simulink model "gru_FL_test"  (R2020a)
settings: Solver=FixedStepAuto  StartTime=0.0  StopTime=Inf  FixedStep=0.001  MaxStep=0.01  RelTol=1e-3
InitFcn:
  | init_gru
StopFcn:
  | %stop_gru
values from neighbouring files (symbols this model uses):
  centro = [points(1); points(2)]    [init_gru.m]
  dir_retta = [1; 0]    [init_gru.m]
  K1 = [1; 1; 1]    [init_gru.m]
  K2 = [0.5; 0.5; 0.5]    [init_gru.m]
  L_ddot_sat = Inf    (= inf)    [init_gru.m]
  L_dot_iniziale = 0    [init_gru.m]
  L_iniziale = z_b_iniziale/cos(theta_iniziale)    [init_gru.m]
  Lsofar = [Lsofar; sum(Lenghts)]    [init_gru.m]
  Ltot = sum(Lenghts)    [init_gru.m]
  n_p = length(points)    [init_gru.m]
  phi_dot_iniziale = 0    [init_gru.m]
  phi_iniziale = 30/180*pi    (= 0.523598775598)    [init_gru.m]
  s_finale = norm(traslazione,2)    [init_gru.m]
  theta_dot_iniziale = 0    [init_gru.m]
  theta_iniziale = 1e-2/180*pi    (= 0.000174532925199)    [init_gru.m]
  theta_rette = [theta_rette ; theta_rette(n_p-2)+pi]    [init_gru.m]
  v_r = v_rif    (= 1)    [init_gru.m]
  x_b_iniziale = 0    [init_gru.m]
  x_t_ddot_sat = Inf    (= inf)    [init_gru.m]
  x_t_dot_iniziale = 0    [init_gru.m]
  x_t_iniziale = x_b_iniziale - L_iniziale * sin(theta_iniziale) * sin(phi_iniziale)    [init_gru.m]
  xp = points(:,1)    [init_gru.m]
  y_b_iniziale = 0    [init_gru.m]
  y_t_ddot_sat = Inf    (= inf)    [init_gru.m]
  y_t_dot_iniziale = 0    [init_gru.m]
  y_t_iniziale = y_b_iniziale - L_iniziale * sin(theta_iniziale) * cos(phi_iniziale)    [init_gru.m]
  yp = points(:,2)    [init_gru.m]
  z_b_iniziale = 2    [init_gru.m]
undefined symbols (not defined in the file or in its folder): indexclot, Lsofarclot, x_M_finale, x_M_iniziale, y_M_finale, y_M_iniziale
libraries: robotcorelib x2, simulink x1
settings Model: Creator=Andrea_Ferroni  LastModifiedBy=Francesco

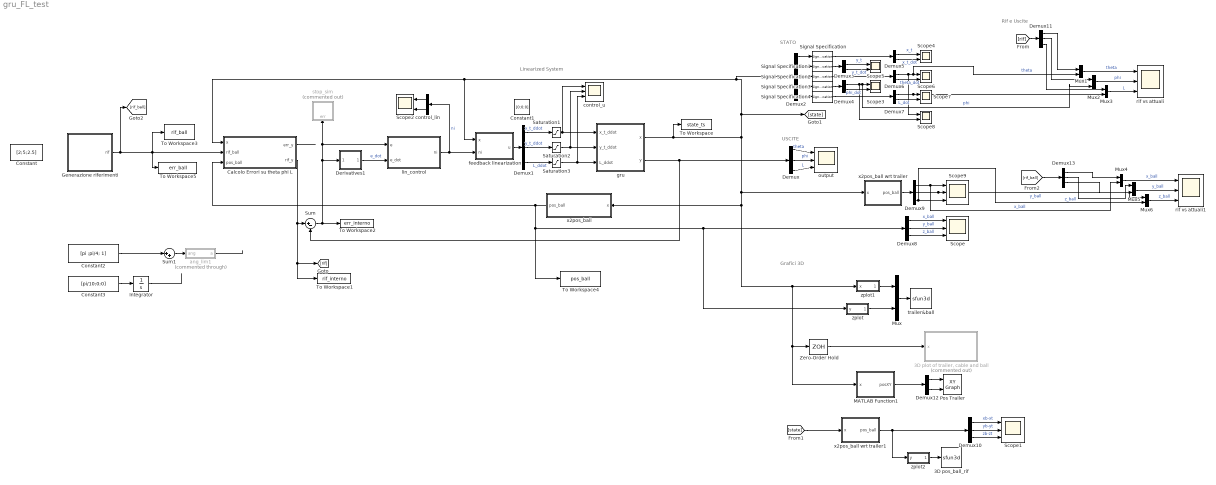
== system gru_FL_test ==
  note: Rif e Uscite
  note: Grafici 3D
  note: USCITE
  note: STATO
  note: Linearized System
  "3D plot of trailer, cable and ball" : MATLAB Function  Commented=on  TreatAsAtomicUnit=on
  3D pos_ball_rif : S-Function  LoadFcn=if exist('sfun3d','file'), sfun3d([],[],[],'LoadBlock'); end  FunctionName=sfun3d  Parameters=ax,T,np,cp,gd,ls,mk,mx,hd,tb  SFunctionDeploymentMode=off  EnableBusSupport=off  mask(3D Graph){np=1, ax=[-50 50 -50 50 -3 3], mx=1e4, T=0.1, cp=[3 2 1], gd=on, hd=off, tb=off, ls=-, mk=none}
      mask prompts: np "Number of moving points (lines)"; ax "Range: [xmin xmax  ymin ymax zmin zmax]"; mx "Max number of points in each line"; T "Sampling Time"; cp "Camera position (use [0 0 1] for 2D XY view)"; gd "Grid (on|off)"; hd "HeadMarkers (on|off)"; tb "Toolbar (on|off)"; ls "LineStyle"; mk "LineMarker"
      mask help:
      | This block plots the position of several points in the XYZ space. The input contains the coordinates of all the points (x1,y1,z1,x2,y2,z2,...).
      | The number of moving points (lines), the XYZ ranges, sampling time, camera position, and grid (among other things) can be set as mask parameters.
      settings: CopyFcn=if exist('sfun3d','file'), sfun3d([],[],[],'CopyBlock'); end  DeleteFcn=if exist('sfun3d','file'), sfun3d([],[],[],'DeleteBlock'); end  NameChangeFcn=if exist('sfun3d','file'), sfun3d([],[],[],'NameChange'); end
      mask Help:
      | This block plots the position of several points in the XYZ space. The input contains the coordinates of all the points (x1,y1,z1,x2,y2,z2,...).
      | The number of moving points (lines), the XYZ ranges, sampling time, camera position, and grid (among other things) can be set as mask parameters.
      mask TypeOptions ls: - | -- | : | -. | none
      mask TypeOptions mk: none | . | + | o | * | x | square | diamond | v | ^ | > | < | pentagram | hexagram
      mask Display: plot([.05 .95 .95 .05 .05],[.45 .45 .95 .95 .45], 0.5+cos(0:0.1:2*pi)*0.3,0.7+sin(0:0.1:2*pi)*0.2)
  Calcolo Errori su theta phi L : MATLAB Function  TreatAsAtomicUnit=on
  Constant : Constant  Value=[2;5;2.5]
  Constant1 : Constant  Value=[0;0;0]
  Constant2 : Constant  Value=[pi ;pi/4; 1]
  Constant3 : Constant  Value=[pi/10;0;0]
  Demux{,1,8..11,13} (7 alike) : Demux  Outputs=3
  Demux{3..7,12} (6 alike) : Demux  Outputs=2
  Demux2 : Demux  Outputs=5
  Derivatives1 : Subsystem
  Generazione riferimenti : Subsystem  Variant=on
  Integrator : Integrator
  MATLAB Function1 : MATLAB Function  TreatAsAtomicUnit=on
  Mux{,1..6} (7 alike) : Mux  Inputs=2
  Pos Trailer : simulink/Sinks/XY Graph  xmin=-100  xmax=100  ymin=-100  ymax=100  st=-1
  Saturation1 : Saturate  UpperLimit=x_t_ddot_sat  LowerLimit=-x_t_ddot_sat
  Saturation2 : Saturate  UpperLimit=y_t_ddot_sat  LowerLimit=-y_t_ddot_sat
  Saturation3 : Saturate  UpperLimit=L_ddot_sat  LowerLimit=-L_ddot_sat
  Scope : Scope  NumInputPorts=3
  Scope1 : Scope  NumInputPorts=3
  Scope{2..8} (7 alike) : Scope  NumInputPorts=2
  Scope9 : Scope  NumInputPorts=3
  Signal Specification{,1..4} (5 alike) : SignalSpecification  Dimensions=[2]
  Sum : Sum  Inputs=|+-
  Sum1 : Sum  Inputs=|++
  To Workspace : ToWorkspace  VariableName=state_ts  SaveFormat=Timeseries  SampleTime=-1
  To Workspace1 : ToWorkspace  VariableName=rif_interno  SaveFormat=Timeseries  SampleTime=-1
  To Workspace2 : ToWorkspace  VariableName=err_interno  SaveFormat=Timeseries  SampleTime=-1
  To Workspace3 : ToWorkspace  VariableName=rif_ball  SaveFormat=Timeseries  SampleTime=-1
  To Workspace4 : ToWorkspace  VariableName=pos_ball  SaveFormat=Timeseries  SampleTime=-1
  To Workspace5 : ToWorkspace  VariableName=err_ball  SaveFormat=Timeseries  SampleTime=-1
  Zero-Order Hold : ZeroOrderHold  SampleTime=1/10
  ang_lim1 : MATLAB Function  Commented=through  TreatAsAtomicUnit=on
  control_lin : Demux  Outputs=2
  control_u : Scope  NumInputPorts=3
  feedback linearization : MATLAB Function  TreatAsAtomicUnit=on
  gru : Subsystem
      mask Display: image('$imagefile'); % Use "Edit Image" on toolstrip to change.
  lin_control : MATLAB Function  TreatAsAtomicUnit=on
  output : Scope  NumInputPorts=3
  rif vs attuali : Scope  NumInputPorts=3
  rif vs attuali1 : Scope  NumInputPorts=3
  stop_sim : Subsystem  Commented=on
  trailer&ball : S-Function  LoadFcn=if exist('sfun3d','file'), sfun3d([],[],[],'LoadBlock'); end  FunctionName=sfun3d  Parameters=ax,T,np,cp,gd,ls,mk,mx,hd,tb  SFunctionDeploymentMode=off  EnableBusSupport=off  mask(3D Graph){np=2, ax=[-50 50 -50 50 -3 3], mx=1e4, T=0.1, cp=[3 2 1], gd=on, hd=off, tb=off, ls=-, mk=none}
      mask prompts: np "Number of moving points (lines)"; ax "Range: [xmin xmax  ymin ymax zmin zmax]"; mx "Max number of points in each line"; T "Sampling Time"; cp "Camera position (use [0 0 1] for 2D XY view)"; gd "Grid (on|off)"; hd "HeadMarkers (on|off)"; tb "Toolbar (on|off)"; ls "LineStyle"; mk "LineMarker"
      mask help:
      | This block plots the position of several points in the XYZ space. The input contains the coordinates of all the points (x1,y1,z1,x2,y2,z2,...).
      | The number of moving points (lines), the XYZ ranges, sampling time, camera position, and grid (among other things) can be set as mask parameters.
      settings: CopyFcn=if exist('sfun3d','file'), sfun3d([],[],[],'CopyBlock'); end  DeleteFcn=if exist('sfun3d','file'), sfun3d([],[],[],'DeleteBlock'); end  NameChangeFcn=if exist('sfun3d','file'), sfun3d([],[],[],'NameChange'); end
      mask Help:
      | This block plots the position of several points in the XYZ space. The input contains the coordinates of all the points (x1,y1,z1,x2,y2,z2,...).
      | The number of moving points (lines), the XYZ ranges, sampling time, camera position, and grid (among other things) can be set as mask parameters.
      mask TypeOptions ls: - | -- | : | -. | none
      mask TypeOptions mk: none | . | + | o | * | x | square | diamond | v | ^ | > | < | pentagram | hexagram
      mask Display: plot([.05 .95 .95 .05 .05],[.45 .45 .95 .95 .45], 0.5+cos(0:0.1:2*pi)*0.3,0.7+sin(0:0.1:2*pi)*0.2)
  x2pos_ball : MATLAB Function  TreatAsAtomicUnit=on
  x2pos_ball wrt trailer : MATLAB Function  TreatAsAtomicUnit=on
  x2pos_ball wrt trailer1 : MATLAB Function  TreatAsAtomicUnit=on
  zplot : MATLAB Function  TreatAsAtomicUnit=on
  zplot1 : MATLAB Function  TreatAsAtomicUnit=on
  zplot2 : MATLAB Function  TreatAsAtomicUnit=on
  wires:
  gru/2(y) -> Sum/2, Demux/1
  lin_control/1(ni) -> control_lin/1, feedback linearization/2(ni)  "ni"
  Derivatives1/1(Out1) -> lin_control/2(e_dot)  "e_dot"
  Demux1/1 -> Saturation1/1  "x_t_ddot"
  Demux1/2 -> Saturation2/1  "y_t_ddot"
  control_lin/2 -> Scope2/2
  control_lin/1 -> Scope2/1
  Demux1/3 -> Saturation3/1  "L_ddot"
  Demux2/1 -> Signal Specification/1
  Demux2/2 -> Signal Specification1/1
  Signal Specification1/1 -> Demux3/1
  Demux2/3 -> Signal Specification2/1
  Demux2/4 -> Signal Specification3/1
  Demux2/5 -> Signal Specification4/1
  Demux3/1 -> Scope5/1  "y_t"
  Demux3/2 -> Scope5/2  "y_t_dot"
  Demux4/1 -> Mux2/2, Scope3/1, Scope8/2  "phi"
  Demux4/2 -> Scope3/2  "phi_dot"
  Signal Specification3/1 -> Demux4/1
  Demux5/1 -> Scope4/1  "x_t"
  Demux5/2 -> Scope4/2  "x_t_dot"
  Signal Specification/1 -> Demux5/1
  Demux6/1 -> Scope8/1, Mux1/2, Scope6/1  "theta"
  Demux6/2 -> Scope6/2  "theta_dot"
  Signal Specification2/1 -> Demux6/1
  Demux7/1 -> Mux3/2, Scope7/1
  Demux7/2 -> Scope7/2  "L_dot"
  Signal Specification4/1 -> Demux7/1
  zplot/1(y_new) -> Mux/2
  Mux/1 -> trailer&ball/1
  zplot1/1(trailer_graph) -> Mux/1
  feedback linearization/1(u) -> Demux1/1
  Demux8/3 -> Scope/3  "z_ball"
  Demux8/2 -> Scope/2  "y_ball"
  Demux8/1 -> Scope/1  "x_ball"
  x2pos_ball wrt trailer/1(pos_ball) -> Demux9/1
  x2pos_ball/1(pos_ball) -> zplot/1(y), Demux8/1, To Workspace4/1, Calcolo Errori su theta phi L/3(pos_ball)
  Demux9/1 -> Mux4/2, Scope9/1  "x_ball"
  Demux9/2 -> Mux5/2, Scope9/2  "y_ball"
  Demux9/3 -> Mux6/2, Scope9/3  "z_ball"
  Sum/1 -> stop_sim/1(err), lin_control/1(e), Derivatives1/1(In1), To Workspace2/1
  Demux/1 -> output/1  "theta"
  Demux/2 -> output/2  "phi"
  Demux/3 -> output/3  "L"
  Demux10/3 -> Scope1/3  "zb-zt"
  Demux10/1 -> Scope1/1  "xb-xt"
  Demux10/2 -> Scope1/2  "yb-yt"
  x2pos_ball wrt trailer1/1(pos_ball) -> zplot2/1(y), Demux10/1
  zplot2/1(y_new) -> 3D pos_ball_rif/1
  Demux11/2 -> Mux2/1
  Demux11/1 -> Mux1/1
  Mux3/1 -> rif vs attuali/3  "L"
  Mux2/1 -> rif vs attuali/2  "phi"
  MATLAB Function1/1(posXY) -> Demux12/1
  Demux12/1 -> Pos Trailer/1
  Demux12/2 -> Pos Trailer/2
  Zero-Order Hold/1 -> "3D plot of trailer, cable and ball"/1(x)
  Saturation1/1 -> control_u/1, gru/1(x_t_ddot)
  Saturation2/1 -> gru/2(y_t_ddot), control_u/2
  Saturation3/1 -> control_u/3, gru/3(L_ddot)
  Demux11/3 -> Mux3/1
  Mux1/1 -> rif vs attuali/1  "theta"
  [rif] -> Demux11/1
  gru/1(x) -> Zero-Order Hold/1, MATLAB Function1/1(x), zplot1/1(x), x2pos_ball/1(x), x2pos_ball wrt trailer/1(x), feedback linearization/1(x), Calcolo Errori su theta phi L/1(x), Demux2/1, [state], To Workspace/1
  [state] -> x2pos_ball wrt trailer1/1(x)
  Sum1/1 -> ang_lim1/1(ang)
  Constant2/1 -> Sum1/1
  Constant3/1 -> Integrator/1
  Integrator/1 -> ?
  Calcolo Errori su theta phi L/1(err_y) -> ?
  Generazione riferimenti/1(rif) -> [rif_ball], To Workspace5/1, To Workspace3/1, Calcolo Errori su theta phi L/2(rif_ball)
  Calcolo Errori su theta phi L/2(rif_y) -> To Workspace1/1, [rif], Sum/1
  ang_lim1/1(a) -> ?
  Mux6/1 -> rif vs attuali1/3  "z_ball"
  Mux4/1 -> rif vs attuali1/1  "x_ball"
  Mux5/1 -> rif vs attuali1/2  "y_ball"
  [rif_ball] -> Demux13/1
  Demux13/1 -> Mux4/1
  Demux13/2 -> Mux5/1
  Demux13/3 -> Mux6/1

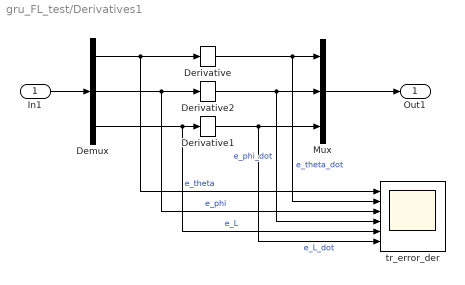
== system gru_FL_test/Derivatives1 ==
  In1 : Inport
  Demux : Demux  Outputs=3
  Derivative : Derivative  CoefficientInTFapproximation=1e10
  Derivative1 : Derivative  CoefficientInTFapproximation=1e10
  Derivative2 : Derivative  CoefficientInTFapproximation=1e10
  Mux : Mux  Inputs=3
  tr_error_der : Scope  NumInputPorts=6
  Out1 : Outport
  wires:
  Mux/1 -> Out1/1
  Demux/2 -> tr_error_der/3, Derivative2/1  "e_phi"
  Derivative/1 -> tr_error_der/2, Mux/1  "e_theta_dot"
  Demux/1 -> tr_error_der/1, Derivative/1  "e_theta"
  In1/1 -> Demux/1
  Derivative2/1 -> tr_error_der/4, Mux/2  "e_phi_dot"
  Demux/3 -> tr_error_der/5, Derivative1/1  "e_L"
  Derivative1/1 -> tr_error_der/6, Mux/3  "e_L_dot"

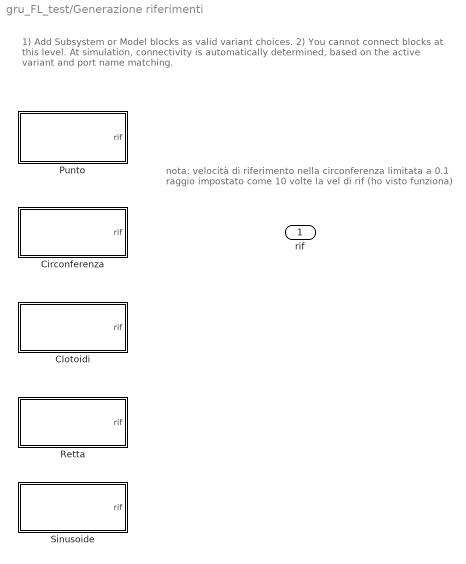
== system gru_FL_test/Generazione riferimenti ==
  note: nota:
      | velocità di riferimento nella circonferenza limitata a 0.1
      | raggio impostato come 10 volte la vel di rif (ho visto funziona)
  note: 1) Add Subsystem or Model blocks as valid variant choices.
      | 2) You cannot connect blocks at this level. At simulation, connectivity is automatically
      | determined, based on the active variant and port name matching.
  Circonferenza : Subsystem  VariantControl=Circonferenza
  Clotoidi : Subsystem  VariantControl=Clotoidi
  Punto : Subsystem  VariantControl=Punto
  Retta : Subsystem  VariantControl=Retta
  Sinusoide : Subsystem  VariantControl=Sinusoide
  rif : Outport

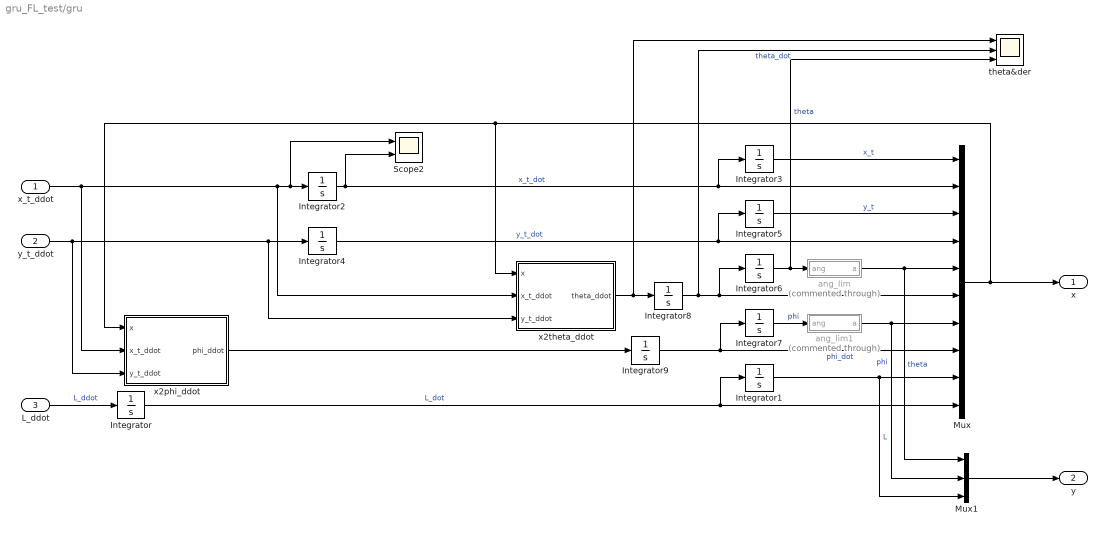
== system gru_FL_test/gru ==
  x_t_ddot : Inport
  y_t_ddot : Inport  Port=2
  L_ddot : Inport  Port=3
  Integrator : Integrator  InitialCondition=L_dot_iniziale
  Integrator1 : Integrator  InitialCondition=L_iniziale
  Integrator2 : Integrator  InitialCondition=x_t_dot_iniziale  UpperSaturationLimit=1e3  LowerSaturationLimit=-1e3
  Integrator3 : Integrator  InitialCondition=x_t_iniziale  LimitOutput=on  UpperSaturationLimit=10  LowerSaturationLimit=-10
  Integrator4 : Integrator  InitialCondition=y_t_dot_iniziale
  Integrator5 : Integrator  InitialCondition=y_t_iniziale  LimitOutput=on  UpperSaturationLimit=10  LowerSaturationLimit=-10
  Integrator6 : Integrator  InitialCondition=theta_iniziale
  Integrator7 : Integrator  InitialCondition=phi_iniziale
  Integrator8 : Integrator  InitialCondition=theta_dot_iniziale
  Integrator9 : Integrator  InitialCondition=phi_dot_iniziale
  Mux : Mux  Inputs=10
  Mux1 : Mux  Inputs=3
  Scope2 : Scope  NumInputPorts=2
  ang_lim : MATLAB Function  Commented=through  TreatAsAtomicUnit=on
  ang_lim1 : MATLAB Function  Commented=through  TreatAsAtomicUnit=on
  theta&der : Scope  NumInputPorts=3
  x2phi_ddot : MATLAB Function  TreatAsAtomicUnit=on
  x2theta_ddot : MATLAB Function  TreatAsAtomicUnit=on
  x : Outport
  y : Outport  Port=2
  wires:
  Integrator3/1 -> Mux/1  "x_t"
  Integrator2/1 -> Scope2/2, Integrator3/1, Mux/2  "x_t_dot"
  Integrator5/1 -> Mux/3  "y_t"
  Integrator4/1 -> Integrator5/1, Mux/4  "y_t_dot"
  Integrator6/1 -> theta&der/3, ang_lim/1(ang)  "theta"
  Integrator8/1 -> theta&der/2, Integrator6/1, Mux/6  "theta_dot"
  Integrator7/1 -> ang_lim1/1(ang)  "phi"
  Integrator9/1 -> Integrator7/1, Mux/8  "phi_dot"
  Integrator1/1 -> Mux1/3, Mux/9  "L"
  L_ddot/1 -> Integrator/1  "L_ddot"
  Integrator/1 -> Integrator1/1, Mux/10  "L_dot"
  x_t_ddot/1 -> x2theta_ddot/2(x_t_ddot), Scope2/1, Integrator2/1, x2phi_ddot/2(x_t_ddot)
  y_t_ddot/1 -> x2theta_ddot/3(y_t_ddot), Integrator4/1, x2phi_ddot/3(y_t_ddot)
  x2theta_ddot/1(theta_ddot) -> theta&der/1, Integrator8/1
  x2phi_ddot/1(phi_ddot) -> Integrator9/1
  Mux/1 -> x2phi_ddot/1(x), x2theta_ddot/1(x), x/1
  ang_lim/1(a) -> Mux1/1, Mux/5  "theta"
  ang_lim1/1(a) -> Mux1/2, Mux/7  "phi"
  Mux1/1 -> y/1

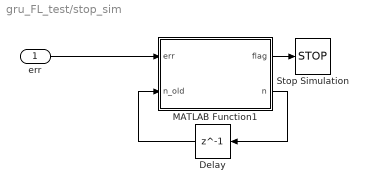
== system gru_FL_test/stop_sim ==
  err : Inport
  Delay : Delay  DelayLength=1
  MATLAB Function1 : MATLAB Function  TreatAsAtomicUnit=on
  Stop Simulation : Stop
  wires:
  MATLAB Function1/2(n) -> Delay/1
  MATLAB Function1/1(flag) -> Stop Simulation/1
  err/1 -> MATLAB Function1/1(err)
  Delay/1 -> MATLAB Function1/2(n_old)

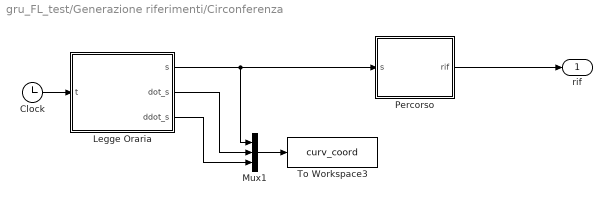
== system gru_FL_test/Generazione riferimenti/Circonferenza ==
  Clock : Clock
  Legge Oraria : MATLAB Function  TreatAsAtomicUnit=on
  Mux1 : Mux  Inputs=3
  Percorso : MATLAB Function  TreatAsAtomicUnit=on
  To Workspace3 : ToWorkspace  VariableName=curv_coord  SaveFormat=Timeseries  SampleTime=-1
  rif : Outport
  wires:
  Legge Oraria/2(dot_s) -> Mux1/2
  Clock/1 -> Legge Oraria/1(t)
  Mux1/1 -> To Workspace3/1
  Legge Oraria/3(ddot_s) -> Mux1/3
  Legge Oraria/1(s) -> Percorso/1(s), Mux1/1
  Percorso/1(rif) -> rif/1

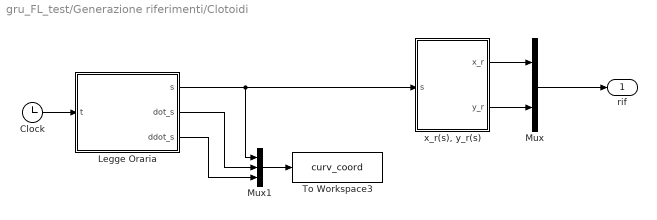
== system gru_FL_test/Generazione riferimenti/Clotoidi ==
  Clock : Clock
  Legge Oraria : MATLAB Function  TreatAsAtomicUnit=on
  Mux : Mux  Inputs=2
  Mux1 : Mux  Inputs=3
  To Workspace3 : ToWorkspace  VariableName=curv_coord  SaveFormat=Timeseries  SampleTime=-1
  "x_r(s), y_r(s)" : MATLAB Function  TreatAsAtomicUnit=on
  rif : Outport
  wires:
  Legge Oraria/1(s) -> Mux1/1, "x_r(s), y_r(s)"/1(s)
  Legge Oraria/2(dot_s) -> Mux1/2
  Clock/1 -> Legge Oraria/1(t)
  Legge Oraria/3(ddot_s) -> Mux1/3
  Mux1/1 -> To Workspace3/1
  "x_r(s), y_r(s)"/2(y_r) -> Mux/2
  "x_r(s), y_r(s)"/1(x_r) -> Mux/1
  Mux/1 -> rif/1

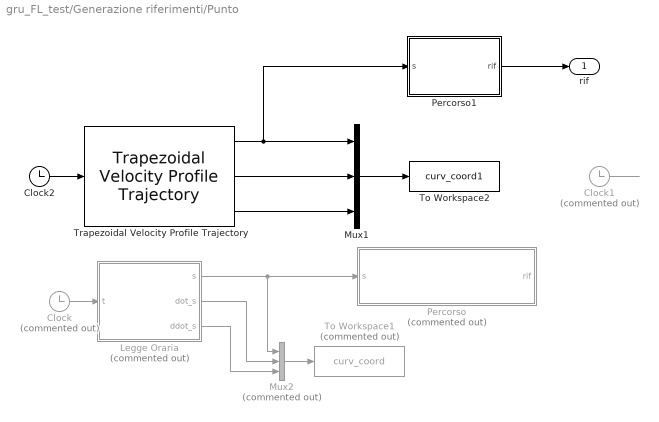
== system gru_FL_test/Generazione riferimenti/Punto ==
  Clock : Clock  Commented=on
  Clock1 : Clock  Commented=on
  Clock2 : Clock
  Legge Oraria : MATLAB Function  Commented=on  TreatAsAtomicUnit=on
  Mux1 : Mux  Inputs=3
  Mux2 : Mux  Commented=on  Inputs=3
  Percorso : MATLAB Function  Commented=on  TreatAsAtomicUnit=on
  Percorso1 : MATLAB Function  TreatAsAtomicUnit=on
  To Workspace1 : ToWorkspace  Commented=on  VariableName=curv_coord  SaveFormat=Timeseries  SampleTime=-1
  To Workspace2 : ToWorkspace  VariableName=curv_coord1  SaveFormat=Timeseries  SampleTime=-1
  Trapezoidal Velocity Profile Trajectory : robotcorelib/Trapezoidal Velocity Profile Trajectory  WaypointSource=Internal  Waypoints="[ 0,  s_finale]"  NumParams=2  Parameter1=Peak Velocity  Parameter2=Acceleration  ParameterSource=Internal  PeakVelocity=v_rif  Acceleration=a_rif  EndTime=[ 1; 1 ]  AccelTime=[ 1; 2 ]  SimulateUsing=Interpreted execution
      settings: SourceProductBaseCode=NV,RO,RR
  rif : Outport
  wires:
  Legge Oraria/2(dot_s) -> Mux2/2
  Clock/1 -> Legge Oraria/1(t)
  Mux2/1 -> To Workspace1/1
  Legge Oraria/3(ddot_s) -> Mux2/3
  Legge Oraria/1(s) -> Mux2/1, Percorso/1(s)
  Trapezoidal Velocity Profile Trajectory/1 -> Percorso1/1(s), Mux1/1
  Trapezoidal Velocity Profile Trajectory/2 -> Mux1/2
  Clock2/1 -> Trapezoidal Velocity Profile Trajectory/1
  Trapezoidal Velocity Profile Trajectory/3 -> Mux1/3
  Clock1/1 -> ?
  Mux1/1 -> To Workspace2/1
  Percorso1/1(rif) -> rif/1

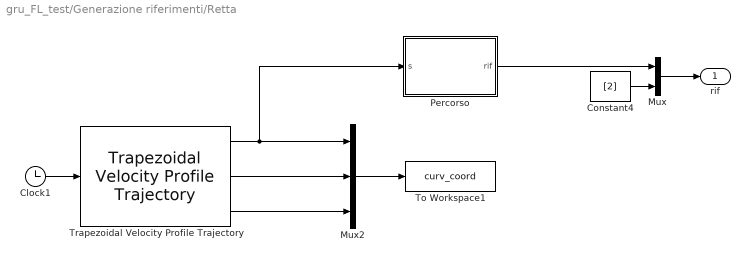
== system gru_FL_test/Generazione riferimenti/Retta ==
  Clock1 : Clock
  Constant4 : Constant  Value=[2]
  Mux : Mux  Inputs=2
  Mux2 : Mux  Inputs=3
  Percorso : MATLAB Function  TreatAsAtomicUnit=on
  To Workspace1 : ToWorkspace  VariableName=curv_coord  SaveFormat=Timeseries  SampleTime=-1
  Trapezoidal Velocity Profile Trajectory : robotcorelib/Trapezoidal Velocity Profile Trajectory  WaypointSource=Internal  Waypoints="[ 0,  1000]"  NumParams=2  Parameter1=Peak Velocity  Parameter2=Acceleration  ParameterSource=Internal  PeakVelocity=v_rif  Acceleration=a_rif  EndTime=[ 1; 1 ]  AccelTime=[ 1; 2 ]  SimulateUsing=Interpreted execution
      settings: SourceProductBaseCode=NV,RO,RR
  rif : Outport
  wires:
  Mux2/1 -> To Workspace1/1
  Clock1/1 -> Trapezoidal Velocity Profile Trajectory/1
  Trapezoidal Velocity Profile Trajectory/1 -> Percorso/1(s), Mux2/1
  Trapezoidal Velocity Profile Trajectory/2 -> Mux2/2
  Trapezoidal Velocity Profile Trajectory/3 -> Mux2/3
  Constant4/1 -> Mux/2
  Mux/1 -> rif/1
  Percorso/1(rif) -> Mux/1

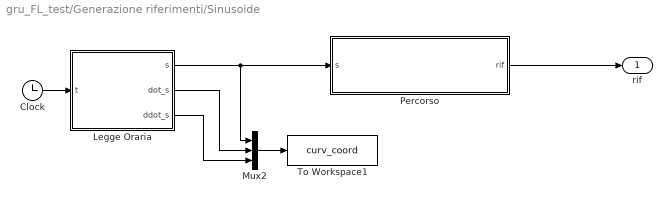
== system gru_FL_test/Generazione riferimenti/Sinusoide ==
  Clock : Clock
  Legge Oraria : MATLAB Function  TreatAsAtomicUnit=on
  Mux2 : Mux  Inputs=3
  Percorso : MATLAB Function  TreatAsAtomicUnit=on
  To Workspace1 : ToWorkspace  VariableName=curv_coord  SaveFormat=Timeseries  SampleTime=-1
  rif : Outport
  wires:
  Legge Oraria/2(dot_s) -> Mux2/2
  Clock/1 -> Legge Oraria/1(t)
  Mux2/1 -> To Workspace1/1
  Legge Oraria/3(ddot_s) -> Mux2/3
  Legge Oraria/1(s) -> Mux2/1, Percorso/1(s)
  Percorso/1(rif) -> rif/1

== matlab function gru_FL_test/gru/x2phi_ddot ==
  data: x input; phi_ddot output; x_t_ddot input; y_t_ddot input
function phi_ddot = fcn(x, x_t_ddot, y_t_ddot)
	
	theta		= x(5);
	theta_dot	= x(6);
	phi			= x(7);
	phi_dot		= x(8);
	L			= x(9);
	L_dot		= x(10);
	
phi_ddot = -2*(L_dot/L)*phi_dot-2*phi_dot*theta_dot*cot(theta) + (-cos(phi)/(sin(theta)*L))*x_t_ddot + (sin(phi)/(sin(theta)*L))*y_t_ddot;

== matlab function gru_FL_test/Generazione riferimenti/Circonferenza/Legge Oraria ==
  data: t input; s output; v_rif parameter; dot_s output; ddot_s output
function [s, dot_s, ddot_s]  = legge_oraria(t, v_rif)
%#codegen PEPO

s = v_rif*t;
dot_s = v_rif;
ddot_s = 0.0;


end

== matlab function gru_FL_test/Generazione riferimenti/Circonferenza/Percorso ==
  data: s input; rif output; centro parameter; v_r parameter
function rif = percorso(s, centro, v_r)

r = 10*v_r;  % 1
theta_circ = s/r;

if theta_circ >=  3*2*pi % dopotre giri ti fermi
	theta_circ = 3*2*pi;
end

rif = centro + r*[cos(theta_circ);sin(theta_circ)];		% circonferenza

end

== matlab function gru_FL_test/Generazione riferimenti/Retta/Percorso ==
  data: s input; rif output; dir_retta parameter; x_b_iniziale parameter; y_b_iniziale parameter
function rif  = retta(s, dir_retta, x_b_iniziale, y_b_iniziale)

rif = [x_b_iniziale;y_b_iniziale] + s * dir_retta;


end

== matlab function gru_FL_test/Generazione riferimenti/Clotoidi/x_r(s), y_r(s) ==
  data: s input; x_r output size=1; y_r output size=1; indexclot parameter; theta_rette parameter; yp parameter; xp parameter; Lsofar parameter; n_p parameter; Lsofarclot parameter; Ltot parameter
function [x_r,y_r] = percorso(s, indexclot, theta_rette, yp, xp, ...
										Lsofar, n_p, Lsofarclot, Ltot)
									
coder.extrinsic('pointsOnClothoid')
% fine percorso
if s >= Ltot
	s = Ltot; % cosi` da plottare l'ultimo punto
end

ntratto=0;
	XYS = [0; 0]; %definito prima

	%Parte per capire in che tratto sono
	if s < Lsofar(1)
		ntratto=1;
	else
		for ii=2:(n_p-1)
			if s>=Lsofar(ii-1) && s<=Lsofar(ii)
				ntratto=ii;
			end
		end
	end	

		%calcolo delle coordinate x e y riferite a s e a ntratto
	if mod(ntratto,2)==1            %tratti dispari - rette
		if ntratto==1
			XYS=[xp(ntratto)+cos(theta_rette(ntratto))*(s); ...
				yp(ntratto)+sin(theta_rette(ntratto))*(s)];
		else
			srel=s-Lsofar(ntratto-1);
			XYS=[	xp(ntratto)	+ cos(theta_rette(ntratto))	* srel; ...
					yp(ntratto)	+ sin(theta_rette(ntratto))	* srel];
		end 

	elseif mod(ntratto,2)==0	%tratti pari - clotoidi
		srel=s-Lsofar(ntratto-1);

		if srel<=Lsofarclot(ntratto/2).Lclot(1)
			XYS = double(pointsOnClothoid( indexclot(ntratto/2).clot.S0, srel ));

		elseif srel>Lsofarclot(ntratto/2).Lclot(1) & srel<=Lsofarclot(ntratto/2).Lclot(2)
			XYS = double(pointsOnClothoid( indexclot(ntratto/2).clot.SM, srel- indexclot(ntratto/2).clot.S0.L ));

		elseif srel>Lsofarclot(ntratto/2).Lclot(2)
			XYS = double(pointsOnClothoid( indexclot(ntratto/2).clot.S1, srel- indexclot(ntratto/2).clot.S0.L - indexclot(ntratto/2).clot.SM.L ));
		end

		%XYS = double(pointsOnClothoid( indexclot(ntratto/2).clot, s-Lsofar(ntratto-1) ));
	end

	x_r = XYS(1);
	y_r = XYS(2);
%--------------------------------------------------
% end function
end

== matlab function gru_FL_test/Generazione riferimenti/Sinusoide/Legge Oraria ==
  data: t input; s output; v_rif parameter; dot_s output; ddot_s output
function [s, dot_s, ddot_s]  = legge_oraria(t, v_rif)
%#codegen PEPO

s = v_rif*t;
dot_s = v_rif;
ddot_s = 0.0;


end

== matlab function gru_FL_test/Generazione riferimenti/Sinusoide/Percorso ==
  data: s input; rif output; dir_retta parameter
function rif  = retta(s, dir_retta)

r = 5;
theta_circ = s/r;

% if theta_circ >=  3*2*pi % dopotre giri ti fermi
% 	theta_circ = 3*2*pi;
% end

rif = dir_retta * s + r*[0; sin(theta_circ)];	% circonferenza

end

== matlab function gru_FL_test/x2pos_ball ==
  data: x input; pos_ball output; z_t parameter
function pos_ball = fcn(x, z_t)
	
	x_t		= x(1);
	y_t		= x(3);
	theta	= x(5);
	phi		= x(7);
	L		= x(9);
	
pos_ball = [x_t + L*sin(theta)*sin(phi); ...
			y_t + L*sin(theta)*cos(phi);...
			z_t + L*cos(theta)];

== matlab function gru_FL_test/x2pos_ball wrt trailer ==
  data: x input; pos_ball output
function pos_ball = fcn(x)
	
	theta	= x(5);
	phi		= x(7);
	L		= x(9);
	
pos_ball = [ L*sin(theta)*sin(phi); ...
			 L*sin(theta)*cos(phi);...
			 L*cos(theta)];

== matlab function gru_FL_test/gru/ang_lim ==
  data: ang input; a output
function a = ang_lim(ang)

	c = cos(ang);
	s = sin(ang);
	a = atan2(s, c);

end

== matlab function gru_FL_test/gru/ang_lim1 ==
  data: ang input; a output
function a = ang_lim(ang)

	c = cos(ang);
	s = sin(ang);
	a = atan2(s, c);

end

== matlab function gru_FL_test/zplot ==
  data: y input; y_new output
function y_new = fcn(y)

y_new	 = y;
y_new(3) = -y_new(3);

end

== matlab function gru_FL_test/zplot1 ==
  data: x input; trailer_graph output; z_t parameter
function trailer_graph = fcn(x, z_t)

	trailer_graph = [x(1); x(3); z_t];

end

== matlab function gru_FL_test/3D plot of trailer, cable and ball ==
  data: x input; z_t parameter
function gru_plot(x, z_t)

coder.extrinsic('plot3')
coder.extrinsic('text')
coder.extrinsic('num2str')

% get relevant signals
x_t		= x(1);
y_t		= x(3);
theta	= x(5);
phi		= x(7);
L		= x(9);

% get mass position
pos_ball = [ L*sin(theta)*sin(phi); ...
			 L*sin(theta)*cos(phi);...
			 -L*cos(theta)];

% figure
figure(1)
plot3(x_t, y_t, -z_t, 'bd', 'MarkerSize', 5)
hold on
plot3(pos_ball(1), pos_ball(2), pos_ball(3), 'ro', 'MarkerSize', 5)
plot3([x_t, pos_ball(1)], [y_t, pos_ball(2)], [-z_t, pos_ball(3)], 'k-', 'LineWidth', 2)
text(0,0,0,['theta ' num2str(theta/pi*180)])
grid on
view([45 10])
xlim([-50 50])
xlabel('X')
ylim([-50 50])
ylabel('Y')
zlim([-3 0.5])
zlabel('Z')
hold off
drawnow

end

== matlab function gru_FL_test/x2pos_ball wrt trailer1 ==
  data: x input; pos_ball output
function pos_ball = fcn(x)
	
	theta	= x(1);
	phi		= x(2);
	L		= x(3);
	
pos_ball = [ L*sin(theta)*sin(phi); ...
			 L*sin(theta)*cos(phi);...
			 L*cos(theta)];

== matlab function gru_FL_test/zplot2 ==
  data: y input; y_new output
function y_new = fcn(y)

y_new	 = y;
y_new(3) = -y_new(3);

end

== matlab function gru_FL_test/MATLAB Function1 ==
  data: x input; z_t parameter; posXY output
function posXY = pos_cart(x, z_t)

posXY = zeros(2,1);
% get relevant signals
posXY(1)		= x(1);
posXY(2)		= x(3);
%pos(3)		= z_t;

end

== matlab function gru_FL_test/ang_lim1 ==
  data: ang input; a output
function a = ang_lim(ang)

	c = cos(ang);
	s = sin(ang);
	a = atan2(s, c);

end

== matlab function gru_FL_test/Generazione riferimenti/Punto/Percorso1 ==
  data: s input; rif output; dir_retta parameter; x_b_iniziale parameter; y_b_iniziale parameter; z_b_iniziale parameter
function rif  = retta(s, dir_retta, x_b_iniziale, y_b_iniziale, z_b_iniziale)

rif = [x_b_iniziale; y_b_iniziale; z_b_iniziale] + s * dir_retta;


end

== matlab function gru_FL_test/Calcolo Errori su theta phi L ==
  data: err_y output; rif_y output; x input; rif_ball input; pos_ball input; z_t parameter
function [err_y, rif_y] = xyrif2err_y(x, rif_ball, pos_ball, z_t)

% Estraiamo i segnali utili
% attuali valori
x_t_now		= x(1);
y_t_now		= x(3);
theta_now	= x(5);
phi_now		= x(7);
L_now		= x(9);
pos_trailer = [x_t_now; y_t_now; z_t];


% err_palla
[theta_rif, phi_rif, L_rif] = pos2out(pos_trailer, rif_ball);
err_theta	= diffang(theta_now, theta_rif);	% theta_rif - theta_now
err_phi		= diffang(phi_now, phi_rif);		% phi_rif - phi_now
err_L		= L_rif - L_now;

% output of function
err_y = [err_theta; err_phi; err_L]; % theta - phi - L
rif_y = [theta_rif; phi_rif; L_rif];


end

%% Extra functions
function [theta, phi, L] = pos2out(pos_trailer, pos_ball)

xb = pos_ball(1);
yb = pos_ball(2);
zb = pos_ball(3);
xt = pos_trailer(1);
yt = pos_trailer(2);
zt = pos_trailer(3);

phi = atan2(xb-xt,yb-yt);

if phi < 1e-3
	theta = atan2(abs(yb-yt), zb-zt);
else
	theta = atan2(abs(xb-xt),(zb-zt)*sin(phi));
end

if abs(theta-pi/2) < 1e-5
	L = norm([xb;yb]-[xt;yt],2);
	
else
	% L = norm(pos_trailer - pos_ball);
	L = abs((zb-zt))/cos(theta);
% 	L = abs(zb-zt);
end

end

% function [theta, phi, L] = pos2out2(pos_trailer, pos_ball)
% 
% xb = pos_ball(1);
% yb = pos_ball(2);
% zb = pos_ball(3);
% xt = pos_trailer(1);
% yt = pos_trailer(2);
% zt = pos_trailer(3);
% 
% L = norm(pos_trailer - pos_ball);
% theta = acos((zb-zt)/L);
% sinphi = (xb-xt)/L*sin(theta);
% cosphi = (yb-yt)/L*sin(theta);
% phi = atan2(sinphi, cosphi);
% 
% end

function ang = diffang( ang1, ang2)

c1 = cos(ang1);
c2 = cos(ang2);
s1 = sin(ang1);
s2 = sin(ang2);

ang = atan2(s2-s1,c2-c1);


end

== matlab function gru_FL_test/lin_control ==
  data: e input; ni output; e_dot input; K1 parameter; K2 parameter
function ni = lin_control(e, e_dot, K1, K2)

ni = K1.*e + K2.*e_dot;
% ni = [0; 0; 0];

end

== matlab function gru_FL_test/feedback linearization ==
  data: x input; ni input; u output
function u = Linearized(x,ni)

	E_inv = inv_E(x);
	G = Gamma(x);
	u =  -E_inv*G + E_inv*ni;

end

% gamma
function Gm = Gamma(x)
	theta		= x(5);
	theta_dot	= x(6);
% 	phi			= x(7);
	phi_dot		= x(8);
	L			= x(9);
	L_dot		= x(10);

Gm =  [(sin(2*theta)*phi_dot^2)/2 - (981*sin(theta))/(100*L) - (2*L_dot*theta_dot)/L;...
                        - 2*phi_dot*theta_dot*cot(theta) - (2*L_dot*phi_dot)/L;...
                                                                             0];

end
% 
function E_in = inv_E(x)
	theta		= x(5);
	phi			= x(7);
	L			= x(9); 



E = [	 -(cos(theta)*sin(phi))/L, -(cos(phi)*cos(theta))/L, 0;...
		 -cos(phi)/(L*sin(theta)),  sin(phi)/(L*sin(theta)), 0;...
								0,                        0, 1];

E_in = inv(E);

end

== matlab function gru_FL_test/Generazione riferimenti/Punto/Legge Oraria ==
  data: t input; s output; v_rif parameter; dot_s output; ddot_s output
function [s, dot_s, ddot_s]  = legge_oraria(t, v_rif)
%#codegen PEPO

s = v_rif*t;
dot_s = v_rif;
ddot_s = 0.0;


end

== matlab function gru_FL_test/gru/x2theta_ddot ==
  data: x input; theta_ddot output; x_t_ddot input; y_t_ddot input; g parameter
function theta_ddot = fcn(x, x_t_ddot, y_t_ddot, g)
	
	theta		= x(5);
	theta_dot	= x(6);
	phi			= x(7);
	phi_dot		= x(8);
	L			= x(9);
	L_dot		= x(10);
	
theta_ddot = -2*(L_dot/L)*theta_dot+0.5*phi_dot^2*sin(2*theta)-(g/L)*sin(theta) + (-cos(theta)*sin(phi)/L)*x_t_ddot + (-cos(theta)*cos(phi)/L)*y_t_ddot;

== matlab function gru_FL_test/stop_sim/MATLAB Function1 ==
  data: flag output; err input; n output; n_old input; threshold parameter
function [flag, n] = stop_function(err, n_old, threshold)
	flag = 0;
	n = n_old;
	if norm(err, 2) < threshold
		n=n+1;
	else
		n=0;
	end
	
	if n > 500
		flag = 1;
		n = 0;
	end
end

== matlab function gru_FL_test/Generazione riferimenti/Punto/Percorso ==
  data: s input; rif output; x_M_finale parameter; x_M_iniziale parameter; y_M_finale parameter; y_M_iniziale parameter
function rif  = punto2punto(s, x_M_finale, x_M_iniziale, y_M_finale, y_M_iniziale)

vett = [x_M_finale - x_M_iniziale; y_M_finale - y_M_iniziale];
Ltot = norm(vett,2);
direzione = vett/Ltot;
offset = 0;

if s >= Ltot
	rif = [x_M_finale + offset; y_M_finale + offset];
else
	rif = [ x_M_iniziale + offset; y_M_iniziale + offset] + s * direzione;
end
% 
% if s > 2*Ltot
% 	s = mod(s, 2*Ltot);
% end
% 
% if s >= Ltot
% 	rif = [ x_M_finale ; y_M_finale ] - (s-Ltot) * direzione;
% 	
% else
% 	rif = [ x_M_iniziale ; y_M_iniziale ] + s * direzione;
% end



end

== matlab function gru_FL_test/Generazione riferimenti/Clotoidi/Legge Oraria ==
  data: t input; s output; v_rif parameter; dot_s output; ddot_s output
function [s, dot_s, ddot_s]  = legge_oraria(t, v_rif)
%#codegen PEPO

s = v_rif*t;
dot_s = v_rif;
ddot_s = 0.0;


end
